simulink model "Writedata_Model"  (R2024b)
settings: Solver=VariableStepAuto  StartTime=0.0  StopTime=10.0  RelTol=1e-3
libraries: NSA_DEVS_LOGISTICS x5, NSA_DEVS_SINKS x3, NSA_DEVS_SOURCES x1
settings Model: Creator=david  LastModifiedBy=peter
settings RTWCC: GPUComputeCapability=3.5

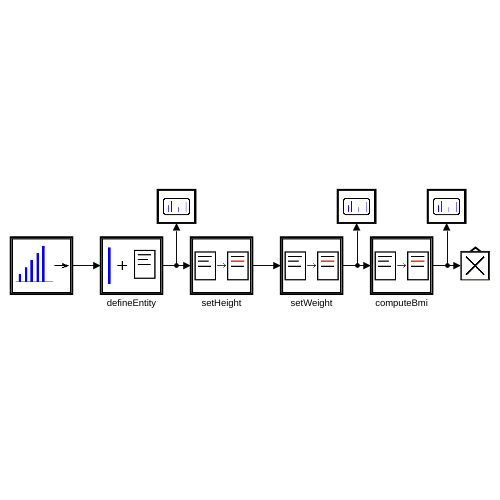
[thumbnail: Simulink's stored preview of the top-level diagram]
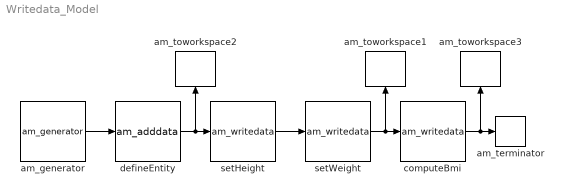
== system Writedata_Model ==
  am_generator : NSA_DEVS_SOURCES/am_generator  tG=1  n0=1  nG=10  tD=[0,2]  debug=0
      settings: SourceProductName=Sources
  am_terminator : NSA_DEVS_LOGISTICS/am_terminator  tau=[0,1]  debug=0
      settings: SourceProductName=Logistics
  am_toworkspace1 : NSA_DEVS_SINKS/am_toworkspace  varname="\"data2Out\""  t0=0  format="\"vector\""  tau=[0,3]  debug=0
      settings: SourceProductName=Sinks
  am_toworkspace2 : NSA_DEVS_SINKS/am_toworkspace  varname="\"data1Out\""  t0=0  format="\"vector\""  tau=[0,3]  debug=0
      settings: SourceProductName=Sinks
  am_toworkspace3 : NSA_DEVS_SINKS/am_toworkspace  varname="\"data3Out\""  t0=0  format="\"vector\""  tau=[0,3]  debug=0
      settings: SourceProductName=Sinks
  computeBmi : NSA_DEVS_LOGISTICS/am_writedata  inFields="[\"height\", \"weight\"]"  outField="\"bmi\""  changeFunc="\"out = in(2)/in(1)^2;\""  tau=[0,1]  debug=0
      settings: SourceProductName=Logistics
  defineEntity : NSA_DEVS_LOGISTICS/am_adddata  fields="[\"name\", \"height\", \"weight\", \"bmi\"]"  values="[\"Peter\", \"1.82\", \"82\", \"0\"]"  numeric=[false, true, true, true]  infield="\"id\""  tau=[0,1]  debug=0
      settings: SourceProductName=Logistics
  setHeight : NSA_DEVS_LOGISTICS/am_writedata  inFields=[]  outField="\"height\""  changeFunc="\"out = 1.78 + 0.08*randn();\""  tau=[0,1]  debug=0
      settings: SourceProductName=Logistics
  setWeight : NSA_DEVS_LOGISTICS/am_writedata  inFields=[]  outField="\"weight\""  changeFunc="\"out = 81 + 8*randn();\""  tau=[0,1]  debug=0
      settings: SourceProductName=Logistics
  wires:
  am_generator/1 -> defineEntity/1
  defineEntity/1 -> setHeight/1, am_toworkspace2/1
  computeBmi/1 -> am_terminator/1, am_toworkspace3/1
  setHeight/1 -> setWeight/1
  setWeight/1 -> computeBmi/1, am_toworkspace1/1
